simulink library "ammclib_bam_S32K3xx"  (R2016a)
(part 11 of 50)

      |           f16C1=2^15-1;
      |           warning(['Parameter f16C1 of ' gcb ' exceeds the fixed-point range.']);
      |         end
      |         if f16C1<-2^15
      |           f16C1=-2^15;
      |           warning(['Parameter f16C1 of ' gcb ' exceeds the fixed-point range.']);
      |         end
      |         if isnan(f16ADCMaxError)
      |           if ~strcmp(f16ADCMaxError_bkup,'0')
      |             set_param(gcb,'f16ADCMaxError','0');
      |           end
      |         else
      |           tmps=num2str(f16ADCMaxError);
      |           if ~strcmp(f16ADCMaxError_bkup,tmps)
      |             set_param(gcb,'f16ADCMaxError',tmps);
      |           end
      |         end
      |         if isnan(f16CC1sc)
      |           if ~strcmp(f16CC1sc_bkup,'0')
      |             set_param(gcb,'f16CC1sc','0');
      |           end
      |         else
      |           tmps=num2str(f16CC1sc);
      |           if ~strcmp(f16CC1sc_bkup,tmps)
      |             set_param(gcb,'f16CC1sc',tmps);
      |           end
      |         end
      |         if isnan(f16CC2sc)
      |           if ~strcmp(f16CC2sc_bkup,'0')
      |             set_param(gcb,'f16CC2sc','0');
      |           end
      |         else
      |           tmps=num2str(f16CC2sc);
      |           if ~strcmp(f16CC2sc_bkup,tmps)
      |             set_param(gcb,'f16CC2sc',tmps);
      |           end
      |         end
      |         if isnan(f16UpperLimit)
      |           if ~strcmp(f16UpperLimit_bkup,'0')
      |             set_param(gcb,'f16UpperLimit','0');
      |           end
      |         else
      |           tmps=num2str(f16UpperLimit);
      |           if ~strcmp(f16UpperLimit_bkup,tmps)
      |             set_param(gcb,'f16UpperLimit',tmps);
      |           end
      |         end
      |         if isnan(f16LowerLimit)
      |           if ~strcmp(f16LowerLimit_bkup,'0')
      |             set_param(gcb,'f16LowerLimit','0');
      |           end
      |         else
      |           tmps=num2str(f16LowerLimit);
      |           if ~strcmp(f16LowerLimit_bkup,tmps)
      |             set_param(gcb,'f16LowerLimit',tmps);
      |           end
      |         end
      |         if isnan(u16NShiftPI)
      |           if ~strcmp(u16NShiftPI_bkup,'0')
      |             set_param(gcb,'u16NShiftPI','0');
      |           end
      |         else
      |           tmps=num2str(u16NShiftPI);
      |           if ~strcmp(u16NShiftPI_bkup,tmps)
      |             set_param(gcb,'u16NShiftPI',tmps);
      |           end
      |         end
      |         if isnan(f16C1)
      |           if ~strcmp(f16C1_bkup,'0')
      |             set_param(gcb,'f16C1','0');
      |           end
      |         else
      |           tmps=num2str(f16C1);
      |           if ~strcmp(f16C1_bkup,tmps)
      |             set_param(gcb,'f16C1',tmps);
      |           end
      |         end
      |         if isnan(u16NShiftI)
      |           if ~strcmp(u16NShiftI_bkup,'0')
      |             set_param(gcb,'u16NShiftI','0');
      |           end
      |         else
      |           tmps=num2str(u16NShiftI);
      |           if ~strcmp(u16NShiftI_bkup,tmps)
      |             set_param(gcb,'u16NShiftI',tmps);
      |           end
      |         end
      |       end
      |     end
      |   catch
      |    warning(['Sample time cannot be calculated for the block ' gcb])
      |   end
      | end
      mask DialogControl timeHint Prompt: Note: Implementation parameters cannot be calculated yet because the block's inherited sample time is unknown. Simulink will update the sample time when you run the simulation.
      mask Display:
      | color('black');
      | pos = get_param(gcb, 'Position');
      | width = pos(3) - pos(1);
      | height = pos(4) - pos(2);
      | tX=width/2;
      | tY=height - 8;
      | color('black');
      | text(tX,tY, 'AMCLIB_Windmilling_F16', 'horizontalAlignment', 'center');
      | if showStates == 2
      |   color('red');
      |   text(tX,tY - 20, ['debugging mode' char(13) char(10) '(limited performance)'], 'horizontalAlignment', 'center');
      | end
